simulink model "Src_0"  (R2026a)
settings: Solver=VariableStepAuto
undefined symbols (not defined in the file): designMultirateFIR
libraries: dspsrcs4 x2, dspmlti4 x1, dspsigops x1
settings Model: Creator=ranja  LastModifiedBy=ranja

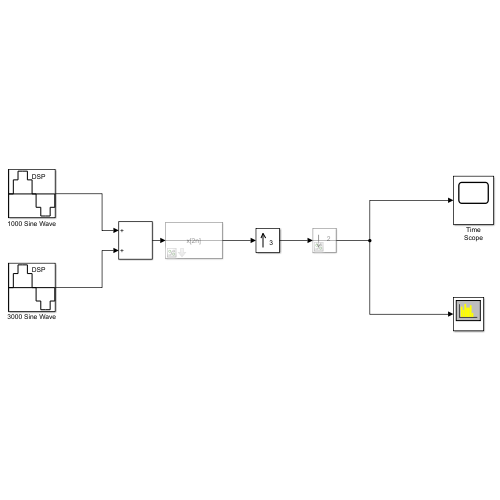
[thumbnail: Simulink's stored preview of the top-level diagram]
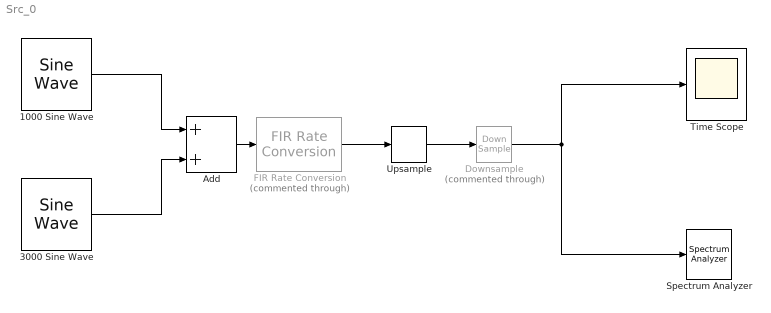
== system Src_0 ==
  1000 Sine Wave : dspsrcs4/Sine Wave  Amplitude=1  Frequency=1000  Phase=0  SampleMode=Discrete  OutComplex=Real  CompMethod=Trigonometric fcn  TableSize=Speed  SampleTime=1/10000  SamplesPerFrame=1000  ResetState=Restart at time zero  OutputFrames=off  dataType=double  wordLen=16  udDataType=sfix(16)  fracBitsMode=Best precision  numFracBits=15  OutDataTypeStr=double  LastOutDataTypeStr=double
  3000 Sine Wave : dspsrcs4/Sine Wave  Amplitude=1  Frequency=3000  Phase=0  SampleMode=Discrete  OutComplex=Real  CompMethod=Trigonometric fcn  TableSize=Speed  SampleTime=1/10000  SamplesPerFrame=1000  ResetState=Restart at time zero  OutputFrames=off  dataType=double  wordLen=16  udDataType=sfix(16)  fracBitsMode=Best precision  numFracBits=15  OutDataTypeStr=double  LastOutDataTypeStr=double
  Add : Sum
  Downsample : DownSample  Commented=through  AllowArbitraryFixedInput=on
  FIR Rate Conversion : dspmlti4/FIR Rate Conversion  Commented=through  FilterSource=Auto  L=1  h=designMultirateFIR(3,2)  M=2  FilterObject=FRC  rateMode=Enforce single-rate processing  AllowArbitraryInputLength=off  roundingMode=Floor  overflowMode=off  firstCoeffDataTypeStr=Inherit: Same word length as input  firstCoeffMin=[]  firstCoeffMax=[]  firstCoeffLastDataTypeStr=Inherit: Same word length as input  outputDataTypeStr=Inherit: Same as accumulator  outputMin=[]  outputMax=[]  outputLastDataTypeStr=Inherit: Same as accumulator
  Spectrum Analyzer : SpectrumAnalyzer  WindowPosition=[368.000000,182.000000,800.000000,500.000000,]  ScopeFrameLocation=window  WindowInvariantSamplesPerUpdate=on  YLimits=[-183.7814 36.4612]
  Time Scope : Scope
      settings: TimeUnits=Metric (based on Time Span)  ActiveDisplayYMinimum=-0.734445375372587  ActiveDisplayYMaximum=1.1627891286883902  YLabel=Amplitude
  Upsample : dspsigops/Upsample  FactorSource=Dialog parameter  UpsamplingFactor=3  MaxUpsamplingFactor=16  SampleOffset=0  InputProcessing=Columns as channels (frame based)  RateOptions=Enforce single-rate processing  InitialConditions=0  mode=Unused parameter value
  wires:
  1000 Sine Wave/1 -> Add/1
  3000 Sine Wave/1 -> Add/2
  Add/1 -> FIR Rate Conversion/1
  Downsample/1 -> Spectrum Analyzer/1, Time Scope/1
  FIR Rate Conversion/1 -> Upsample/1
  Upsample/1 -> Downsample/1
